simulink model "Proyecto"  (R2022a)
settings: Solver=VariableStepAuto  StartTime=0.0  StopTime=10.0  RelTol=1e-3
undefined symbols (not defined in the file or in its folder): B, I, lc, lm, mb, wb, wc, wm
settings Model: Creator=Joseph  LastModifiedBy=Joseph

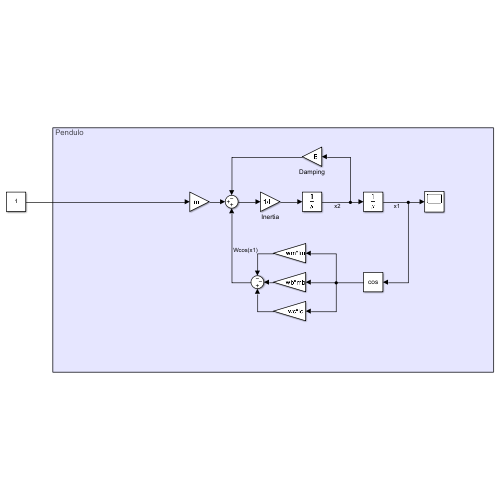
[thumbnail: Simulink's stored preview of the top-level diagram]
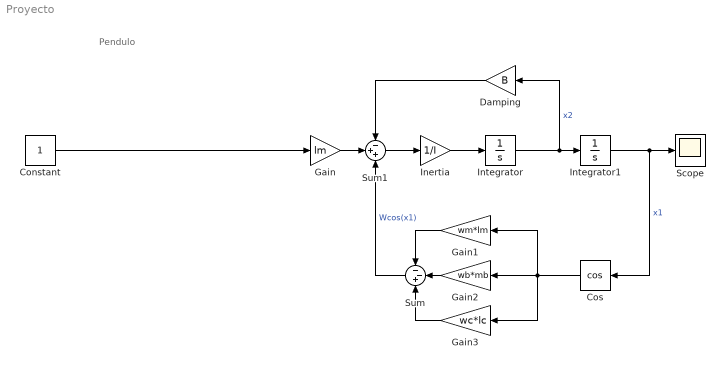
== system Proyecto ==
  note: Pendulo
  Constant : Constant
  Cos : Trigonometry  Operator=cos
  Damping : Gain  Gain=B
  Gain : Gain  Gain=lm
  Gain1 : Gain  Gain=wm*lm
  Gain2 : Gain  Gain=wb*mb
  Gain3 : Gain  Gain=wc*lc
  Inertia : Gain  Gain=1/I
  Integrator : Integrator  ZeroCross=off
  Integrator1 : Integrator  ZeroCross=off
  Scope : Scope
  Sum : Sum  Inputs=--+
  Sum1 : Sum  Inputs=-++
  wires:
  Integrator/1 -> Damping/1, Integrator1/1  "x2"
  Integrator1/1 -> Cos/1, Scope/1  "x1"
  Cos/1 -> Gain1/1, Gain3/1, Gain2/1
  Gain1/1 -> Sum/1
  Gain2/1 -> Sum/2
  Gain3/1 -> Sum/3
  Sum/1 -> Sum1/3  "Wcos(x1)"
  Damping/1 -> Sum1/1
  Gain/1 -> Sum1/2
  Sum1/1 -> Inertia/1
  Inertia/1 -> Integrator/1
  Constant/1 -> Gain/1
